simulink model "DFIG_BESS_In_power_LFnetwork_5bus"  (R2017b)
settings: Solver=ode23tb  StartTime=0.0  StopTime=10  MaxStep=0.04  RelTol=1e-3  EnableMultiTasking=on
values from neighbouring files (symbols this model uses):
  beta = beta (k)    [Parameter_2M_DFIG_BESS.m]
  Cbus = 80e-3    (= 0.08)    [Parameter_2M_DFIG_BESS.m]
  Cbus_bess = 15e-3    (= 0.015)    [Parameter_2M_DFIG_BESS.m]
  Cfilter = 80e-3    (= 0.08)    [Parameter_2M_DFIG_BESS.m]
  cp_opt_abs = abs(max(Cp))    [Parameter_2M_DFIG_BESS.m]
  D = 0.1    [Parameter_2M_DFIG_BESS.m]
  f = 60    [Parameter_2M_DFIG_BESS.m]
  Fs = 1.8    [Parameter_2M_DFIG_BESS.m]
  fsw = 4e3    (= 4000)    [Parameter_2M_DFIG_BESS.m]
  J = 90    [Parameter_2M_DFIG_BESS.m]
  ki_id = (wni^2)*Lr*sigma    (= 491.599501999)    [Parameter_2M_DFIG_BESS.m]
  ki_idg = (wnig^2)*Lg    (= 68.6450725305)    [Parameter_2M_DFIG_BESS.m]
  ki_iq = ki_id    (= 491.599501999)    [Parameter_2M_DFIG_BESS.m]
  ki_iqg = ki_idg    (= 68.6450725305)    [Parameter_2M_DFIG_BESS.m]
  ki_v = -300000    [Parameter_2M_DFIG_BESS.m]
  kp_id = (2*wni*sigma*Lr)-Rr    (= 0.5771)    [Parameter_2M_DFIG_BESS.m]
  kp_idg = (2*wnig*Lg)-Rg    (= 0.364153420404)    [Parameter_2M_DFIG_BESS.m]
  kp_iq = kp_id    (= 0.5771)    [Parameter_2M_DFIG_BESS.m]
  kp_iqg = kp_idg    (= 0.364153420404)    [Parameter_2M_DFIG_BESS.m]
  kp_v = -1000    [Parameter_2M_DFIG_BESS.m]
  Kpg = 1/(1.5*Vs*sqrt(2/3))    [Parameter_2M_DFIG_BESS.m]
  Kqg = -Kpg    [Parameter_2M_DFIG_BESS.m]
  lambda_opt = abs(lambda(posicion))    [Parameter_2M_DFIG_BESS.m]
  Lfilter = 483e-6    (= 0.000483)    [Parameter_2M_DFIG_BESS.m]
  Lg = 483e-6    (= 0.000483)    [Parameter_2M_DFIG_BESS.m]
  Lm = 2.5e-3    (= 0.0025)    [Parameter_2M_DFIG_BESS.m]
  Lr = Lm + Lsr    (= 0.002587)    [Parameter_2M_DFIG_BESS.m]
  Ls = Lm + Lsi    (= 0.002587)    [Parameter_2M_DFIG_BESS.m]
  Lsi = 87e-6    (= 8.7e-05)    [Parameter_2M_DFIG_BESS.m]
  n = 1800    [Parameter_2M_DFIG_BESS.m]
  N = 100    [Parameter_2M_DFIG_BESS.m]
  p = 2    [Parameter_2M_DFIG_BESS.m]
  Ps = 2e6    (= 2000000)    [Parameter_2M_DFIG_BESS.m]
  Radio = 44    [Parameter_2M_DFIG_BESS.m]
  Rfilter = 20e-3    (= 0.02)    [Parameter_2M_DFIG_BESS.m]
  ro = 1.225    [Parameter_2M_DFIG_BESS.m]
  Rr = 2.9e-3    (= 0.0029)    [Parameter_2M_DFIG_BESS.m]
  Rs = 2.6e-3    (= 0.0026)    [Parameter_2M_DFIG_BESS.m]
  sigma = 1- Lm^2/(Ls*Lr)    (= 0.0661284179513)    [Parameter_2M_DFIG_BESS.m]
  Vbus_ref = 1200    [Parameter_2M_DFIG_BESS.m]
  Vdc_bat_ref = 1300    [Parameter_2M_DFIG_BESS.m]
  Vs = 690    [Parameter_2M_DFIG_BESS.m]
undefined symbols (not defined in the file or in its folder): D1, Delta, DiscIntNeverNeededParam, Ion, Lithium, sigbuilder_block
libraries: powerlib x69, powerlib_meascontrol x21, electricdrivelib x1, peGeneralControl x1
(part 2 of 3)

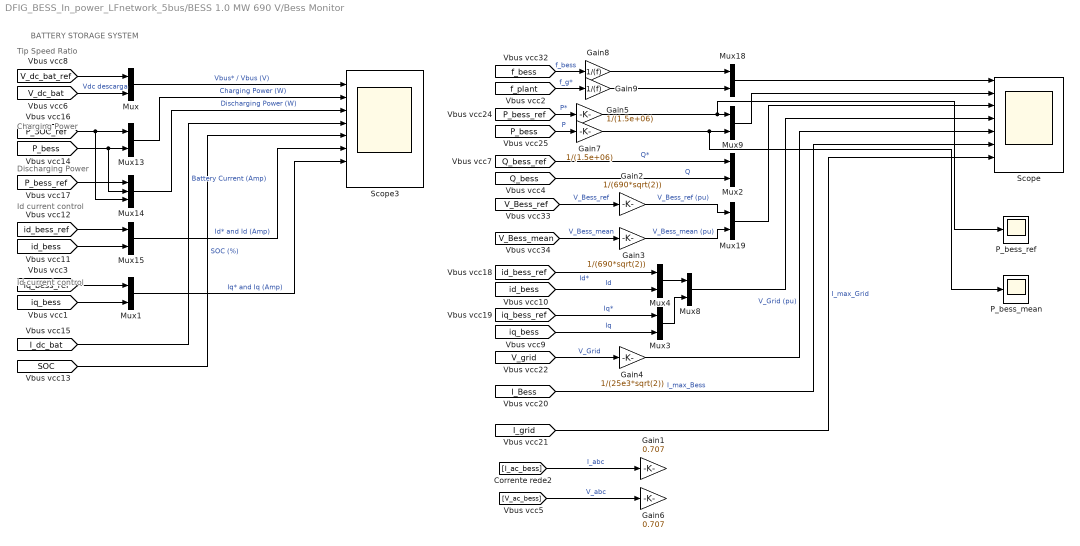
== system DFIG_BESS_In_power_LFnetwork_5bus/BESS 1.0 MW 690 V/Bess Monitor ==
  note: BATTERY STORAGE SYSTEM
  note: Tip Speed Ratio
  note: Charging Power
  note: Discharging Power
  note: Id current control
  note: Id current control
  Gain1 : Gain  Gain=0.707
  Gain2 : Gain  Gain=1/(690*sqrt(2))
  Gain3 : Gain  Gain=1/(690*sqrt(2))
  Gain4 : Gain  Gain=1/(25e3*sqrt(2))
  Gain5 : Gain  Gain=1/(1.5e+06)
  Gain6 : Gain  Gain=0.707
  Gain7 : Gain  Gain=1/(1.5e+06)
  Gain8 : Gain  Gain=1/(f)
  Gain9 : Gain  Gain=1/(f)
  Mux{,1..4,8..9,13,15,18..19} (11 alike) : Mux  Inputs=2
  Mux14 : Mux  Inputs=3
  P_bess_mean : Scope
  P_bess_ref : Scope
  Scope : Scope  NumInputPorts=8
  Scope3 : Scope  NumInputPorts=8
  wires:
  [P_bess_ref] -> Mux14/1
  Mux13/1 -> Scope3/2  "Charging Power (W)"
  [P_SOC_ref] -> Mux14/3, Mux13/1
  [P_bess] -> Mux14/2, Mux13/2
  [id_bess_ref] -> Mux15/1
  [V_dc_bat_ref] -> Mux/1
  Mux/1 -> Scope3/1  "Vbus* / Vbus (V)"
  [id_bess] -> Mux15/2
  Mux14/1 -> Scope3/3  "Discharging Power (W)"
  [SOC] -> Scope3/5  "SOC (%)"
  [I_dc_bat] -> Scope3/4  "Battery Current (Amp)"
  Mux15/1 -> Scope3/6  "Id* and Id (Amp)"
  [V_dc_bat] -> Mux/2  "Vdc descarga"
  [iq_bess] -> Mux1/2
  [iq_bess_ref] -> Mux1/1
  Mux1/1 -> Scope3/7  "Iq* and Iq (Amp)"
  [Q_bess_ref] -> Mux2/1  "Q*"
  [iq_bess_ref] -> Mux3/1  "Iq*"
  [id_bess] -> Mux4/2  "Id"
  [iq_bess] -> Mux3/2  "Iq"
  [id_bess_ref] -> Mux4/1  "Id*"
  Mux4/1 -> Mux8/1
  Mux3/1 -> Mux8/2
  [P_bess_ref] -> Gain5/1  "P*"
  [f_bess] -> Gain8/1  "f_bess"
  [f_plant] -> Gain9/1  "f_g*"
  Mux18/1 -> Scope/1
  [V_Bess_ref] -> Gain2/1  "V_Bess_ref"
  [V_Bess_mean] -> Gain3/1  "V_Bess_mean"
  [V_ac_bess] -> Gain6/1  "V_abc"
  [I_ac_bess] -> Gain1/1  "I_abc"
  [V_grid] -> Gain4/1  "V_Grid"
  [P_bess] -> Gain7/1  "P"
  [Q_bess] -> Mux2/2  "Q"
  Gain2/1 -> Mux19/1  "V_Bess_ref (pu)"
  Gain3/1 -> Mux19/2  "V_Bess_mean (pu)"
  Gain4/1 -> Scope/5  "V_Grid (pu)"
  [I_Bess] -> Scope/6  "I_max_Bess"
  [I_grid] -> Scope/7  "I_max_Grid"
  Mux9/1 -> Scope/2
  Mux19/1 -> Scope/3
  Mux8/1 -> Scope/4
  Gain5/1 -> P_bess_ref/1, Mux9/1
  Gain7/1 -> P_bess_mean/1, Mux9/2
  Gain8/1 -> Mux18/1
  Gain9/1 -> Mux18/2

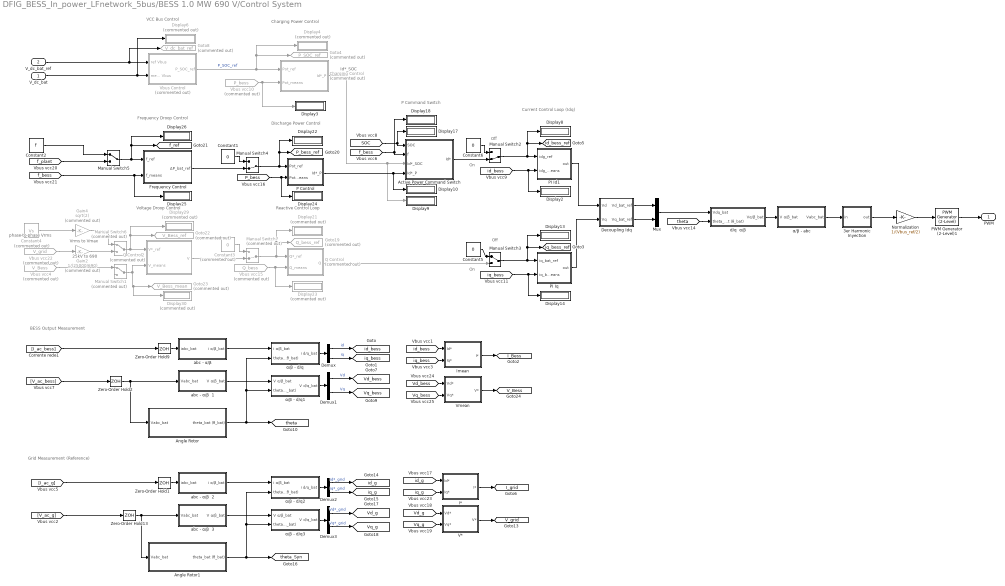
== system DFIG_BESS_In_power_LFnetwork_5bus/BESS 1.0 MW 690 V/Control System ==
  note: BESS Output Measurement
  note: Id*_SOC
  note: Grid Measurement (Reference)
  note: Current Control Loop (Idq)
  note: Discharge Power Control
  note: Frequency Droop Control
  note: Voltage Droop Control
  note: Reactive Control Loop
  note: 25kV to 690
  note: VCC Bus Control
  note: Charging Power Control
  note: P Command Switch
  note: Vrms to Vmax
  note: phase-to-phase Vrms
  note: On
  note: Off
  note: On
  note: Off
  V_dc_bat : Inport
  V_dc_bat_ref : Inport  Port=2
  " Angle Rotor" : Subsystem
  " Angle Rotor1" : Subsystem
  3er Harmonic Inyection : Subsystem
  Active Power Command Switch : Subsystem
  Charging Control : Subsystem  Commented=on
  Constant1 : Constant  Value=0
  Constant2 : Constant  Value=f
  Constant3 : Constant  Commented=on  Value=0
  Constant4 : Constant  Commented=on  Value=Vs
  Constant5 : Constant  Value=0
  Constant6 : Constant  Value=0
  Decoupling Idq : Subsystem
  Demux{,1..3} (4 alike) : Demux  Outputs=2
  Display{2..3,8..10,13..14,17..18,22,24..26} (13 alike) : Display
  Display{4,6,21,23,29..30} (6 alike) : Display  Commented=on
  Frequency Control : Subsystem
  Gain2 : Gain  Commented=on  Gain=1/(25000/690)
  Gain4 : Gain  Commented=on  Gain=sqrt(2)
  Goto19 : Goto  Commented=on  GotoTag=Q_bess_ref  TagVisibility=global
  Goto22 : Goto  Commented=on  GotoTag=V_Bess_ref  TagVisibility=global
  Goto23 : Goto  Commented=on  GotoTag=V_Bess_mean  TagVisibility=global
  Goto4 : Goto  Commented=on  GotoTag=P_SOC_ref  TagVisibility=global
  Goto8 : Goto  Commented=on  GotoTag=V_dc_bat_ref  TagVisibility=global
  I* : Subsystem
  Imean : Subsystem
  Manual Switch1 : ManualSwitch  Commented=on
  Manual Switch2 : ManualSwitch  CurrentSetting=0
  Manual Switch3 : ManualSwitch
  Manual Switch4 : ManualSwitch  CurrentSetting=0
  Manual Switch5 : ManualSwitch
  Manual Switch6 : ManualSwitch  Commented=on
  Manual Switch7 : ManualSwitch  Commented=on  CurrentSetting=0
  Mux : Mux  Inputs=2
  Normalization : Gain  Gain=1/(Vbus_ref/2)
  P Control : Subsystem
  PI Id1 : Subsystem
  PI Iq : Subsystem
  PWM Generator (2-Level)1 : powerlib_meascontrol/Pulse & Signal Generators/PWM Generator (2-Level)  ModulatorType=Three-phase bridge (6 pulses)  ModulatorMode=Unsynchronized  Fc=fsw  Pc=0  nF=27  MinMax="[ -1  1 ]"  SamplingTechnique=Natural  ModulatingSignals=off  m=0.8  Freq=60  Phase=0  Ts=0  ShowCarrierOutport=off
      settings: SourceProductName=Simscape Power Systems
  Q Control : Subsystem  Commented=on
  Q Control2 : Subsystem  Commented=on
  V* : Subsystem
  Vbus Control : Subsystem  Commented=on
  Vbus vcc10 : From  Commented=on  GotoTag=P_bess  TagVisibility=global
  Vbus vcc15 : From  Commented=on  GotoTag=Q_bess  TagVisibility=global
  Vbus vcc22 : From  Commented=on  GotoTag=V_grid  TagVisibility=global
  Vbus vcc4 : From  Commented=on  GotoTag=V_Bess  TagVisibility=global
  Vmean : Subsystem
  Zero-Order Hold{1..2,9,13} (4 alike) : ZeroOrderHold  SampleTime=1/fsw
  "abc - α/β  " : Subsystem
  abc - α/β  1 : Subsystem
  abc - α/β  2 : Subsystem
  abc - α/β  3 : Subsystem
  "d/q  α/β " : Subsystem
  α/β - abc : Subsystem
  α/β - d/q : Subsystem
  α/β - d/q1 : Subsystem
  α/β - d/q2 : Subsystem
  α/β - d/q3 : Subsystem
  PWM : Outport
  tag scope: I_Bess=global, I_grid=global, P_bess_ref=global, V_Bess=global, V_grid=global, Vd_bess=global, Vd_g=global, Vq_bess=global, Vq_g=global, f_ref=global, id_bess=global, id_bess_ref=global, id_g=global, iq_bess=global, iq_bess_ref=global, iq_g=global, theta=global, theta_Syn=global
  wires:
  PWM Generator (2-Level)1/1 -> PWM/1
  α/β - d/q/1(i d/q_bat) -> Demux/1
  Zero-Order Hold2/1 -> " Angle Rotor"/1(Vabc_bat), abc - α/β  1/1(Vabc_bat)
  α/β - abc/1(Vabc_bat) -> 3er Harmonic Inyection/1(in)
  Zero-Order Hold9/1 -> "abc - α/β  "/1(iabc_bat)
  "d/q  α/β "/1("Vα/β_bat ") -> α/β - abc/1(V α/β_bat)
  "abc - α/β  "/1(i α/β_bat) -> α/β - d/q/1(i α/β_bat)
  3er Harmonic Inyection/1(out) -> Normalization/1
  PI Id1/1(out) -> Decoupling Idq/1(Vd)
  PI Iq/1("out ") -> Decoupling Idq/2(Vq)
  Normalization/1 -> PWM Generator (2-Level)1/1
  V_dc_bat/1 -> Display6/1, Vbus Control/2("means Vbus ")
  [f_bess] -> Active Power Command Switch/2(f), Display18/1
  [SOC] -> Active Power Command Switch/1(SOC), Display17/1
  V_dc_bat_ref/1 -> Goto8/1, Vbus Control/1("ref Vbus ")
  Vbus Control/1(P_SOC_ref) -> Goto4/1, Display4/1, Charging Control/1("Pot_ref ")  "P_SOC_ref"
  Vbus vcc10/1 -> Charging Control/2("Pot_means "), Display3/1
  Demux1/1 -> [Vd_bess]  "Vd"
  abc - α/β  1/1(V α/β_bat) -> α/β - d/q1/1(V α/β_bat)
  α/β - d/q1/1(V d/q_bat) -> Demux1/1
  Demux1/2 -> [Vq_bess]  "Vq"
  Mux/1 -> "d/q  α/β "/1(Vdq_bat)
  Decoupling Idq/1(" Vd_bat_ref") -> Mux/1
  Decoupling Idq/2(" Vq_bat_ref") -> Mux/2
  " Angle Rotor"/1(theta_bat (θ_bat)) -> α/β - d/q1/2(theta_bat (θ_bat)), α/β - d/q/2(theta_bat (θ_bat)), [theta]
  Demux/1 -> [id_bess]  "id"
  Demux/2 -> [iq_bess]  "iq"
  [theta] -> "d/q  α/β "/2(theta_bat (θ_bat))
  [id_bess] -> PI Id1/2(idg_means), Display2/1
  [iq_bess] -> Display14/1, PI Iq/2(iq_bat_means)
  Demux3/2 -> [Vq_g]  "Vq*_grid"
  Demux3/1 -> [Vd_g]  "Vd*_grid"
  abc - α/β  3/1(V α/β_bat) -> α/β - d/q3/1(V α/β_bat)
  abc - α/β  2/1(i α/β_bat) -> α/β - d/q2/1(i α/β_bat)
  " Angle Rotor1"/1(theta_bat (θ_bat)) -> α/β - d/q3/2(theta_bat (θ_bat)), α/β - d/q2/2(theta_bat (θ_bat)), [theta_Syn]
  Demux2/1 -> [id_g]  "id*_grid"
  Demux2/2 -> [iq_g]  "iq*_grid"
  α/β - d/q2/1(i d/q_bat) -> Demux2/1
  α/β - d/q3/1(V d/q_bat) -> Demux3/1
  [I_ac_g] -> Zero-Order Hold1/1
  [V_ac_g] -> Zero-Order Hold13/1
  Zero-Order Hold1/1 -> abc - α/β  2/1(iabc_bat)
  Zero-Order Hold13/1 -> " Angle Rotor1"/1(Vabc_bat), abc - α/β  3/1(Vabc_bat)
  [P_bess] -> Display24/1, P Control/2("Pot_means ")
  Manual Switch2/1 -> Display8/1, [id_bess_ref], PI Id1/1(idg_ref)
  Manual Switch3/1 -> Display13/1, [iq_bess_ref], PI Iq/1(iq_bat_ref)
  [f_bess] -> Display25/1, Frequency Control/2(f_means)
  Manual Switch4/1 -> [P_bess_ref], Display22/1, P Control/1("Pot_ref ")
  Frequency Control/1("ΔP_bat_ref ") -> Manual Switch4/2
  Constant1/1 -> Manual Switch4/1
  Manual Switch5/1 -> Display26/1, [f_ref], Frequency Control/1(f_ref)
  [Vq_g] -> V*/2(Vq*)
  [Vd_g] -> V*/1(Vd*)
  [Vd_bess] -> Vmean/1(Vd*)
  [Vq_bess] -> Vmean/2(Vq*)
  Vbus vcc15/1 -> Display23/1, Q Control/2(Q_means)
  Manual Switch7/1 -> Goto19/1, Display21/1, Q Control/1(Q*_ref)
  Constant3/1 -> Manual Switch7/1
  [f_plant] -> Manual Switch5/2
  Constant2/1 -> Manual Switch5/1
  Constant5/1 -> Manual Switch3/1
  Q Control2/1("V ") -> Manual Switch7/2
  V*/1("V* ") -> [V_grid]
  Vmean/1("V* ") -> [V_Bess]
  Manual Switch6/1 -> Q Control2/1(V*_ref), Display29/1, Goto22/1
  [I_ac_bess] -> Zero-Order Hold9/1
  [V_ac_bess] -> Zero-Order Hold2/1
  Vbus vcc22/1 -> Gain2/1
  Gain2/1 -> Manual Switch6/2
  Q Control/1("Q ") -> Manual Switch3/2
  Active Power Command Switch/1(Id*) -> Manual Switch2/2
  Charging Control/1(Id*_P) -> Display9/1, Active Power Command Switch/3(Id*_SOC)
  P Control/1(Id*_P) -> Active Power Command Switch/4(Id*_P), Display10/1
  Constant4/1 -> Gain4/1
  Gain4/1 -> Manual Switch6/1
  Imean/1("I* ") -> [I_Bess]
  [iq_bess] -> Imean/2(Iq*)
  [id_bess] -> Imean/1(Id*)
  I*/1("I* ") -> [I_grid]
  [id_g] -> I*/1(Id*)
  [iq_g] -> I*/2(Iq*)
  Constant6/1 -> Manual Switch2/1
  Manual Switch1/1 -> Q Control2/2(V_means), Display30/1, Goto23/1
  Vbus vcc4/1 -> Manual Switch1/1

== system DFIG_BESS_In_power_LFnetwork_5bus/BESS 1.0 MW 690 V/Measurement of Power - Frequency ==
  FP : Fcn  Commented=on  Expr=cos(atan(u[1]/u[2]))
  Manual Switch3 : ManualSwitch
  Mux : Mux  Commented=on  Inputs=2
  PLL (3ph)1 : powerlib_meascontrol/PLL/PLL (3ph)  Commented=on  Fmin=45  Par_Init=[0, f]  ParK=[180, 3200, 1]  TcD=1e-4  MaxRateChangeFreq=12  FilterCutOffFreq=25  Ts=0  AGC=on
  "Power (3ph, Instantaneous)1" : powerlib_meascontrol/Measurements/Power (3ph, Instantaneous)
      settings: SourceProductName=Simscape Power Systems
  Scope : Scope  Commented=on
  F (Hz) : Outport
  P (W) : Outport  Port=2
  Q (VAR) : Outport  Port=3
  Angle (0) : Outport  Port=4
  tag scope: P_bess=global, Q_bess=global, f_bess=global, wt_mean=global
  wires:
  [V_ac_bess] -> "Power (3ph, Instantaneous)1"/1, PLL (3ph)1/1
  "Power (3ph, Instantaneous)1"/1 -> [P_bess], Mux/2, P (W)/1  "Pot"
  [I_ac_bess] -> "Power (3ph, Instantaneous)1"/2
  "Power (3ph, Instantaneous)1"/2 -> Mux/1, Q (VAR)/1, [Q_bess]
  PLL (3ph)1/2 -> Angle (0)/1, [wt_mean]
  Mux/1 -> FP/1
  FP/1 -> Scope/1
  [f_dfig_bess] -> Manual Switch3/1
  PLL (3ph)1/1 -> Manual Switch3/2
  Manual Switch3/1 -> F (Hz)/1, [f_bess]

== system DFIG_BESS_In_power_LFnetwork_5bus/BESS 1.0 MW 690 V/Subsystem1 ==
  In1 : Inport
  Bus Selector : BusSelector  OutputSignals=SOC (%),Current (A),Voltage (V)
  tag scope: I_dc_bat=global, SOC=global, V_dc_bat=global
  wires:
  Bus Selector/3 -> [V_dc_bat]  "<Voltage (V)>"
  Bus Selector/1 -> [SOC]  "<SOC (%)>"
  In1/1 -> Bus Selector/1
  Bus Selector/2 -> [I_dc_bat]  "<Current (A)>"

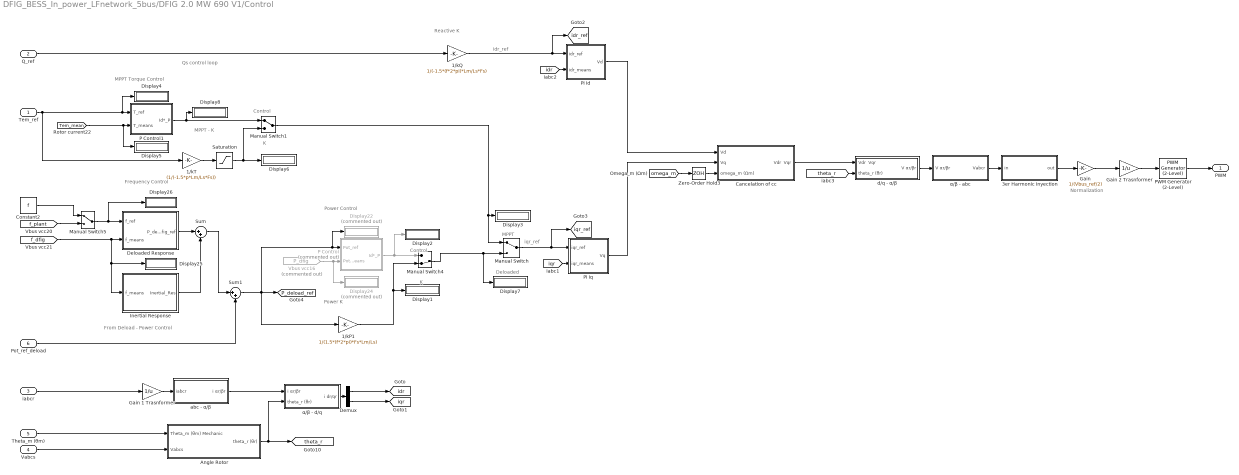
== system DFIG_BESS_In_power_LFnetwork_5bus/DFIG 2.0 MW 690 V1/Control ==
  note: Normalization
  note: iqr_ref
  note: idr_ref
  note: Qs control loop
  note: Reactive K
  note: MPPT - K
  note: From Deload - Power Control
  note: Frequency Control
  note: Power Control
  note: Power K
  note: MPPT
  note: Deloaded
  note: Control
  note: K
  note: MPPT Torque Control
  note: Control
  note: K
  Tem_ref : Inport
  Q_ref : Inport  Port=2
  iabcr : Inport  Port=3
  Vabcs : Inport  Port=4
  Theta_m (θm) : Inport  Port=5
  Pot_ref_deload : Inport  Port=6
  " Angle Rotor" : Subsystem
  1/kP1 : Gain  Gain=1/(1.5*(f*2*pi)*Fs*Lm/Ls)
  1/kQ : Gain  Gain=1/(-1.5*(f*2*pi)*Lm/Ls*Fs)
  1/kT : Gain  Gain=(1/(-1.5*p*Lm/Ls*Fs))
  3er Harmonic Inyection : Subsystem
  Cancelation of cc : Subsystem
  Constant2 : Constant  Value=f
  Deloaded Response : Subsystem
  Demux : Demux  Outputs=2
  Display{1..8,25..26} (10 alike) : Display
  Display22 : Display  Commented=on
  Display24 : Display  Commented=on
  Gain : Gain  Gain=1/(Vbus_ref/2)
  Gain 1 Trasnformer : Gain  Gain=1/u
  Gain 2 Trasnformer : Gain  Gain=1/u
  Inertial Response : Subsystem
  Manual Switch : ManualSwitch
  Manual Switch1 : ManualSwitch
  Manual Switch4 : ManualSwitch  CurrentSetting=0
  Manual Switch5 : ManualSwitch
  P Control : Subsystem  Commented=on
  P Control1 : Subsystem
  PI Id : Subsystem
  PI Iq : Subsystem
  PWM Generator (2-Level) : powerlib_meascontrol/Pulse & Signal Generators/PWM Generator (2-Level)  ModulatorType=Three-phase bridge (6 pulses)  ModulatorMode=Unsynchronized  Fc=fsw  Pc=0  nF=27  MinMax="[ -1  1 ]"  SamplingTechnique=Natural  ModulatingSignals=off  m=0.8  Freq=60  Phase=0  Ts=0  ShowCarrierOutport=off
      settings: SourceProductName=Simscape Power Systems
  Saturation : Saturate  UpperLimit=3500  LowerLimit=0
  Sum : Sum  Inputs=|++
  Sum1 : Sum  Inputs=|++
  Vbus vcc16 : From  Commented=on  GotoTag=P_dfig  TagVisibility=global
  Zero-Order Hold3 : ZeroOrderHold  SampleTime=1/fsw
  "abc - α/β " : Subsystem
  d/q - α/β : Subsystem
  α/β - abc : Subsystem
  α/β - d/q : Subsystem
  PWM : Outport
  tag scope: P_deload_ref=global, idr=global, idr_ref=global, iqr=global, iqr_ref=global, theta_r=global
  wires:
  α/β - abc/1(Vabcr) -> 3er Harmonic Inyection/1(in)
  d/q - α/β/1(V αr/βr) -> α/β - abc/1(V αr/βr)
  iabcr/1 -> Gain 1 Trasnformer/1
  "abc - α/β "/1(i αr/βr) -> α/β - d/q/1(i αr/βr)
  3er Harmonic Inyection/1(out) -> Gain/1
  Theta_m (θm)/1 -> " Angle Rotor"/1(Theta_m (θm) Mechanic)
  Vabcs/1 -> " Angle Rotor"/2(Vabcs)
  " Angle Rotor"/1(theta_r (θr)) -> [theta_r], α/β - d/q/2(theta_r (θr))
  PI Id/1(Vd) -> Cancelation of cc/1(Vd)
  PI Iq/1(Vq) -> Cancelation of cc/2(Vq)
  α/β - d/q/1(i dr/qr) -> Demux/1
  Demux/2 -> [iqr]
  Demux/1 -> [idr]
  Q_ref/1 -> 1/kQ/1
  Cancelation of cc/1(Vdr  Vqr) -> d/q - α/β/1(Vdr  Vqr)
  Gain/1 -> Gain 2 Trasnformer/1
  Gain 1 Trasnformer/1 -> "abc - α/β "/1(iabcr)
  Gain 2 Trasnformer/1 -> PWM Generator (2-Level)/1
  PWM Generator (2-Level)/1 -> PWM/1
  1/kQ/1 -> [idr_ref], PI Id/1(idr_ref)
  Manual Switch/1 -> [iqr_ref], PI Iq/1(iqr_ref)
  [idr] -> PI Id/2(idr_means)
  [iqr] -> PI Iq/2(iqr_means)
  Constant2/1 -> Manual Switch5/1
  [f_dfig] -> Inertial Response/1(f_means), Display25/1, Deloaded Response/2(f_means)
  Manual Switch5/1 -> Display26/1, Deloaded Response/1(f_ref)
  [f_plant] -> Manual Switch5/2
  [theta_r] -> d/q - α/β/2(theta_r (θr))
  [omega_m] -> Zero-Order Hold3/1
  Zero-Order Hold3/1 -> Cancelation of cc/3(omega_m (Ωm))
  Deloaded Response/1("P_deloaded_dfig_ref ") -> Sum/1
  Sum/1 -> Sum1/1
  Pot_ref_deload/1 -> Sum1/2
  Inertial Response/1("Inertial_Res ") -> Sum/2
  Vbus vcc16/1 -> Display24/1, P Control/2("Pot_means ")
  Sum1/1 -> 1/kP1/1, [P_deload_ref], Display22/1, P Control/1("Pot_ref ")
  P Control/1(Id*_P) -> Manual Switch4/1, Display2/1
  1/kP1/1 -> Display1/1, Manual Switch4/2
  Manual Switch4/1 -> Display7/1, Manual Switch/2
  1/kT/1 -> Saturation/1
  P Control1/1(Id*_P) -> Display8/1, Manual Switch1/1
  Manual Switch1/1 -> Display3/1, Manual Switch/1
  Tem_ref/1 -> Display4/1, P Control1/1("T_ref "), 1/kT/1
  [Tem_mean] -> Display5/1, P Control1/2("T_means ")
  Saturation/1 -> Display6/1, Manual Switch1/2

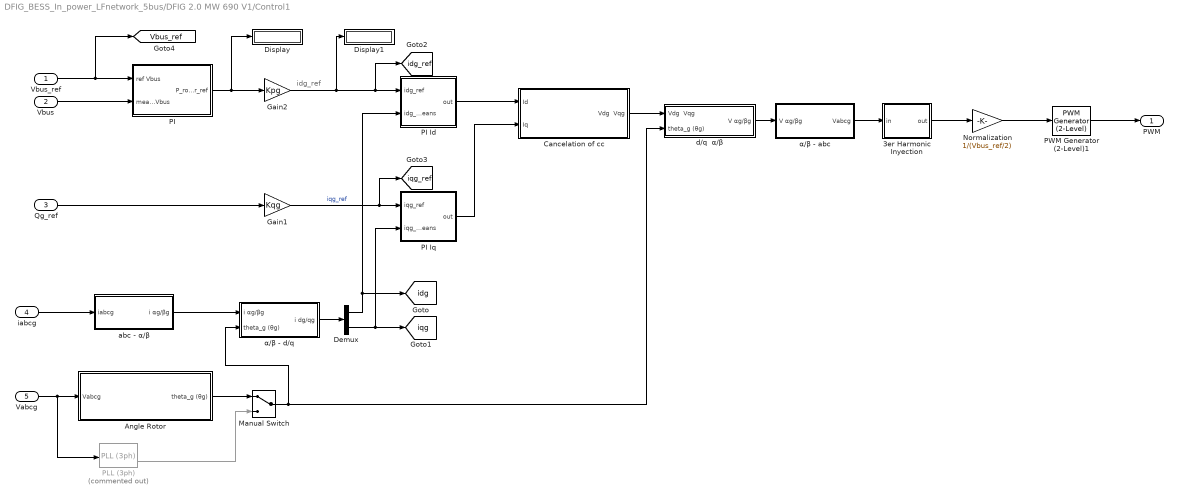
== system DFIG_BESS_In_power_LFnetwork_5bus/DFIG 2.0 MW 690 V1/Control1 ==
  note: idg_ref
  Vbus_ref : Inport
  Vbus : Inport  Port=2
  Qg_ref : Inport  Port=3
  iabcg : Inport  Port=4
  "Vabcg " : Inport  Port=5
  " Angle Rotor" : Subsystem
  3er Harmonic Inyection : Subsystem
  Cancelation of cc : Subsystem
  Demux : Demux  Outputs=2
  Display : Display
  Display1 : Display
  Gain1 : Gain  Gain=Kqg
  Gain2 : Gain  Gain=Kpg
  Manual Switch : ManualSwitch
  Normalization : Gain  Gain=1/(Vbus_ref/2)
  PI : Subsystem
  PI Id : Subsystem
  PI Iq : Subsystem
  PLL (3ph) : powerlib_meascontrol/PLL/PLL (3ph)  Commented=on  Fmin=45  Par_Init=[0, 60]  ParK=[180, 3200, 1]  TcD=1e-4  MaxRateChangeFreq=12  FilterCutOffFreq=25  Ts=0  AGC=on
      link override Model/abc to dq0: Alignment=Aligned with phase A axis
  PWM Generator (2-Level)1 : powerlib_meascontrol/Pulse & Signal Generators/PWM Generator (2-Level)  ModulatorType=Three-phase bridge (6 pulses)  ModulatorMode=Unsynchronized  Fc=fsw  Pc=0  nF=27  MinMax="[ -1  1 ]"  SamplingTechnique=Natural  ModulatingSignals=off  m=0.8  Freq=60  Phase=0  Ts=0  ShowCarrierOutport=off
      settings: SourceProductName=Simscape Power Systems
  "abc - α/β  " : Subsystem
  "d/q  α/β " : Subsystem
  α/β - abc : Subsystem
  α/β - d/q : Subsystem
  PWM : Outport
  tag scope: Vbus_ref=global, idg=global, idg_ref=global, iqg=global, iqg_ref=global
  wires:
  Normalization/1 -> PWM Generator (2-Level)1/1
  Cancelation of cc/1(Vdg  Vqg) -> "d/q  α/β "/1(Vdg  Vqg)
  Gain1/1 -> PI Iq/1(iqg_ref), [iqg_ref]  "iqg_ref"
  Demux/1 -> PI Id/2(idg_means), [idg]
  Demux/2 -> PI Iq/2(iqg_means), [iqg]
  PI Iq/1(out) -> Cancelation of cc/2(Iq)
  PI Id/1(out) -> Cancelation of cc/1(Id)
  3er Harmonic Inyection/1(out) -> Normalization/1
  "abc - α/β  "/1(i αg/βg) -> α/β - d/q/1(i αg/βg)
  "d/q  α/β "/1(V αg/βg) -> α/β - abc/1(V αg/βg)
  iabcg/1 -> "abc - α/β  "/1(iabcg)
  Vbus_ref/1 -> [Vbus_ref], PI/1("ref Vbus ")
  Gain2/1 -> Display1/1, [idg_ref], PI Id/1(idg_ref)
  Vbus/1 -> PI/2("means Vbus ")
  Qg_ref/1 -> Gain1/1
  α/β - abc/1(Vabcg) -> 3er Harmonic Inyection/1(in)
  "Vabcg "/1 -> " Angle Rotor"/1("Vabcg "), PLL (3ph)/1
  PI/1(P_rotor_ref) -> Display/1, Gain2/1
  " Angle Rotor"/1(theta_g (θg)) -> Manual Switch/1
  Manual Switch/1 -> "d/q  α/β "/2(theta_g (θg)), α/β - d/q/2(theta_g (θg))
  α/β - d/q/1(i dg/qg) -> Demux/1
  PLL (3ph)/2 -> Manual Switch/2
  PWM Generator (2-Level)1/1 -> PWM/1

== system DFIG_BESS_In_power_LFnetwork_5bus/DFIG 2.0 MW 690 V1/Deload ==
  Wind speed (m/s) : Inport
  CP : Constant  Value=0.40
  CP1 : Constant  Value=0.44
  Display1 : Display
  Display2 : Display
  Mux6 : Mux  Inputs=2
  Mux7 : Mux  Inputs=2
  Pt_deload : Fcn  Expr=0.5*ro*pi*(Radio)^2*(u[1])^3*u[2]
  Pt_max : Fcn  Expr=0.5*ro*pi*(Radio)^2*(u[1])^3*u[2]
  Scope1 : Scope  NumInputPorts=2
  Sum : Sum  Inputs=|-+
  P_deload : Outport
  P_Max : Outport  Port=2
  P_backup : Outport  Port=3
  wires:
  CP/1 -> Mux6/2
  Mux6/1 -> Pt_deload/1
  Wind speed (m/s)/1 -> Mux7/1, Mux6/1
  Mux7/1 -> Pt_max/1
  CP1/1 -> Mux7/2
  Pt_deload/1 -> Sum/1, Display2/1, Scope1/1, P_deload/1
  Pt_max/1 -> Sum/2, P_Max/1, Display1/1, Scope1/2
  Sum/1 -> P_backup/1

== system DFIG_BESS_In_power_LFnetwork_5bus/DFIG 2.0 MW 690 V1/MPPT ==
  note: Zone 2: MPPT with Vw 5 - 11
  Omega_m : Inport
  Display1 : Display
  Display2 : Display
  Display3 : Display
  Gearbox Ratio Generator Torque (-)1 : Gain  Gain=-1/N
  Gearbox Ratio1 : Gain  Gain=1/N
  Kopt : Gain  Gain=0.5*ro*pi*(Radio)^5/(lambda_opt)^3*cp_opt_abs
  Product2 : Product  Inputs=**  SaturateOnIntegerOverflow=on  InputSameDT=on  OutDataTypeStr=Inherit: Same as first input
  Saturation : Saturate  UpperLimit=2.6e+06  LowerLimit=0
  omega^2 : Fcn  Expr=(u[1])^2
  Tem_ref : Outport
  "Pot_ref " : Outport  Port=2
  wires:
  Gearbox Ratio1/1 -> Product2/2, omega^2/1
  omega^2/1 -> Kopt/1
  Kopt/1 -> Product2/1, Display3/1, Gearbox Ratio Generator Torque (-)1/1
  Product2/1 -> Saturation/1, Display1/1  "Pt"
  Gearbox Ratio Generator Torque (-)1/1 -> Display2/1, Tem_ref/1
  Omega_m/1 -> Gearbox Ratio1/1
  Saturation/1 -> "Pot_ref "/1

== system DFIG_BESS_In_power_LFnetwork_5bus/DFIG 2.0 MW 690 V1/Measurement of Power - Frequency ==
  FP : Fcn  Commented=on  Expr=cos(atan(u[1]/u[2]))
  Manual Switch3 : ManualSwitch
  Mux : Mux  Commented=on  Inputs=2
  PLL (3ph)1 : powerlib_meascontrol/PLL/PLL (3ph)  Commented=on  Fmin=45  Par_Init=[0, f]  ParK=[180, 3200, 1]  TcD=1e-4  MaxRateChangeFreq=12  FilterCutOffFreq=25  Ts=0  AGC=on
  "Power (3ph, Instantaneous)1" : powerlib_meascontrol/Measurements/Power (3ph, Instantaneous)
      settings: SourceProductName=Simscape Power Systems
  Scope : Scope  Commented=on
  F (Hz) : Outport
  P (W) : Outport  Port=2
  Q (VAR) : Outport  Port=3
  Angle (0) : Outport  Port=4
  tag scope: P_dfig=global, Q_dfig=global, f_dfig=global, wt_mean_dfig=global
  wires:
  [Vdfig] -> "Power (3ph, Instantaneous)1"/1, PLL (3ph)1/1
  "Power (3ph, Instantaneous)1"/1 -> Mux/2, P (W)/1, [P_dfig]  "Pot"
  [Idfig] -> "Power (3ph, Instantaneous)1"/2
  "Power (3ph, Instantaneous)1"/2 -> Mux/1, Q (VAR)/1, [Q_dfig]
  PLL (3ph)1/2 -> Angle (0)/1, [wt_mean_dfig]
  Mux/1 -> FP/1
  FP/1 -> Scope/1
  [f_dfig_bess] -> Manual Switch3/1
  Manual Switch3/1 -> [f_dfig], F (Hz)/1
  PLL (3ph)1/1 -> Manual Switch3/2

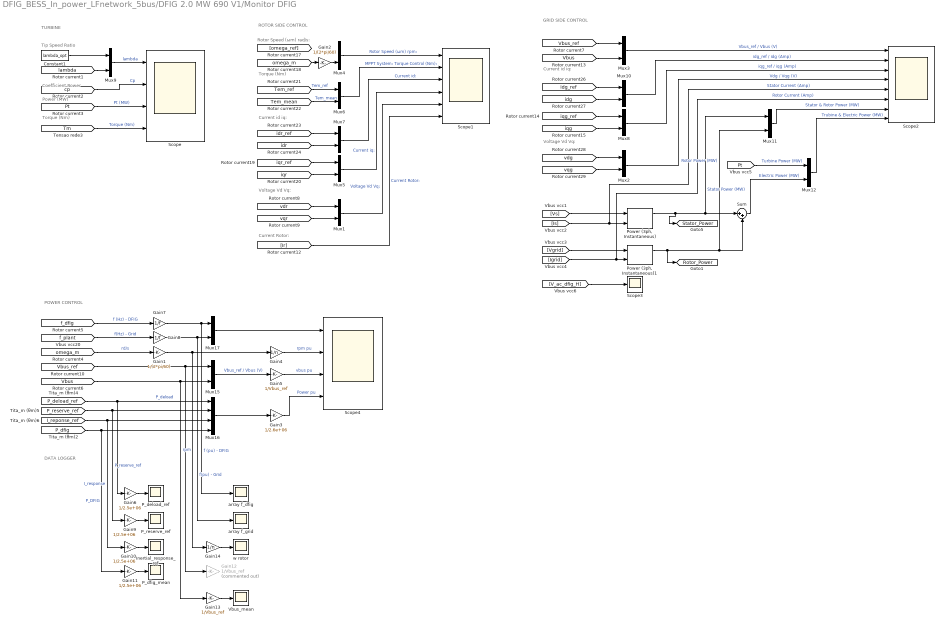
== system DFIG_BESS_In_power_LFnetwork_5bus/DFIG 2.0 MW 690 V1/Monitor DFIG ==
  note: ROTOR SIDE CONTROL
  note: Torque (Nm)
  note: Current id iq:
  note: Rotor Speed (ωm) rad/s:
  note: Voltage Vd Vq:
  note: TURBINE
  note: Torque (Nm)
  note: Power (MW)
  note: Coefficient Power
  note: Tip Speed Ratio
  note: GRID SIDE CONTROL
  note: Current id iq:
  note: Voltage Vd Vq:
  note: Current Rotor:
  note: POWER CONTROL
  note: DATA LOGGER
  Constant1 : Constant  Value=lambda_opt
  Gain1 : Gain  Gain=1/(2*pi/60)
  Gain{6,9..11} (4 alike) : Gain  Gain=1/2.5e+06
  Gain12 : Gain  Commented=on  Gain=1/Vbus_ref
  Gain13 : Gain  Gain=1/Vbus_ref
  Gain14 : Gain  Gain=1/n
  Gain2 : Gain  Gain=1/(2*pi/60)
  Gain3 : Gain  Gain=1/2.6e+06
  Gain4 : Gain  Gain=1/n
  Gain5 : Gain  Gain=1/Vbus_ref
  Gain7 : Gain  Gain=1/f
  Gain8 : Gain  Gain=1/f
  Inertial_response_ref : Scope
  Mux{1..12,15,17} (14 alike) : Mux  Inputs=2
  Mux16 : Mux
  P_deload_ref : Scope
  P_dfig_mean : Scope
  P_reserve_ref : Scope
  "Power (3ph, Instantaneous)" : powerlib_meascontrol/Measurements/Power (3ph, Instantaneous)
      settings: SourceProductName=Simscape Power Systems
  "Power (3ph, Instantaneous)1" : powerlib_meascontrol/Measurements/Power (3ph, Instantaneous)
      settings: SourceProductName=Simscape Power Systems
  Scope : Scope  NumInputPorts=4
  Scope1 : Scope  NumInputPorts=6
  Scope2 : Scope  NumInputPorts=8
  Scope3 : Scope
  Scope4 : Scope  NumInputPorts=4
  Sum : Sum  Inputs=|++
  Vbus_mean : Scope
  array f_dfig : Scope
  array f_grid : Scope
  w rotor : Scope
  tag scope: Rotor_Power=global, Stator_Power=global
  wires:
  [iqr_ref] -> Mux5/1
  [iqr] -> Mux5/2
  [idr] -> Mux7/2
  [idr_ref] -> Mux7/1
  [vdr] -> Mux1/1
  [vqr] -> Mux1/2
  [vqg] -> Mux2/2
  [vdg] -> Mux2/1
  [idg_ref] -> Mux10/1
  [idg] -> Mux10/2
  [iqg] -> Mux8/2
  [iqg_ref] -> Mux8/1
  [Tem_ref] -> Mux6/1  "Tem_ref"
  [Vbus] -> Mux3/2
  [Vbus_ref] -> Mux3/1
  [cp] -> Scope/2  "Cp"
  [Pt] -> Scope/3  "Pt (MW)"
  [Tm] -> Scope/4  "Torque (Nm)"
  Mux4/1 -> Scope1/1  "Rotor Speed (ωm) rpm:"
  Mux6/1 -> Scope1/2  "MPPT System: Torque Control (Nm):"
  Mux7/1 -> Scope1/3  "Current id:"
  Mux5/1 -> Scope1/4  "Current iq:"
  Mux1/1 -> Scope1/5  "Voltage Vd Vq:"
  [Ir] -> Scope1/6  "Current Rotor:"
  [omega_m] -> Gain2/1
  Gain2/1 -> Mux4/2
  Mux3/1 -> Scope2/1  "Vbus_ref / Vbus (V)"
  Mux10/1 -> Scope2/2  "idg_ref / idg (Amp)"
  Mux8/1 -> Scope2/3  "iqg_ref / iqg (Amp)"
  Mux2/1 -> Scope2/4  "Vdg / Vqg (V)"
  [lambda] -> Mux9/2
  Constant1/1 -> Mux9/1
  Mux9/1 -> Scope/1  "lambda"
  [Tem_mean] -> Mux6/2  "Tem_mean"
  [Vs] -> "Power (3ph, Instantaneous)"/1
  [Vgrid] -> "Power (3ph, Instantaneous)1"/1
  [Igrid] -> "Power (3ph, Instantaneous)1"/2, Scope2/6  "Rotor Current (Amp)"
  [Is] -> "Power (3ph, Instantaneous)"/2, Scope2/5  "Stator Current (Amp)"
  "Power (3ph, Instantaneous)"/1 -> [Stator_Power], Mux11/1, Sum/1  "Stator Power (MW)"
  "Power (3ph, Instantaneous)1"/1 -> [Rotor_Power], Sum/2, Mux11/2  "Rotor Power (MW)"
  Sum/1 -> Mux12/2  "Electric Power (MW)"
  Mux11/1 -> Scope2/7  "Stator & Rotor Power (MW)"
  [Pt] -> Mux12/1  "Turbine Power (MW)"
  Mux12/1 -> Scope2/8  "Trubine & Electric Power (MW)"
  [V_ac_dfig_H] -> Scope3/1
  [omega_m] -> Gain1/1  "rd/s"
  [Vbus] -> Gain13/1, Mux15/2
  [Vbus_ref] -> Gain12/1, Mux15/1
  [P_deload_ref] -> Gain6/1, Mux16/1  "P_deload"
  [P_reserve_ref] -> Gain9/1, Mux16/2  "P_reserve_ref"
  [I_reponse_ref] -> Gain10/1, Mux16/3  "I_response"
  Mux17/1 -> Scope4/1
  [f_dfig] -> Gain7/1  "f (Hz) - DFIG"
  [f_plant] -> Gain8/1  "f(Hz) - Grid"
  Gain1/1 -> Gain14/1, Gain4/1  "rpm"
  Mux15/1 -> Gain5/1  "Vbus_ref / Vbus (V)"
  [P_dfig] -> Gain11/1, Mux16/4  "P_DFIG"
  Gain4/1 -> Scope4/2  "rpm pu"
  Gain5/1 -> Scope4/3  "vbus pu"
  Mux16/1 -> Gain3/1
  Gain7/1 -> array f_dfig/1, Mux17/1  "f (pu) - DFIG"
  Gain8/1 -> array f_grid/1, Mux17/2  "f(pu) - Grid"
  Gain3/1 -> Scope4/4  "Power pu"
  Gain6/1 -> P_deload_ref/1
  Gain9/1 -> P_reserve_ref/1
  Gain10/1 -> Inertial_response_ref/1
  Gain11/1 -> P_dfig_mean/1
  Gain13/1 -> Vbus_mean/1
  Gain14/1 -> w rotor/1

== system DFIG_BESS_In_power_LFnetwork_5bus/DFIG 2.0 MW 690 V1/Signal Builder ==
  Demux : Demux  Tag=STV Demux  Outputs=1
  FromWs : FromWorkspace  Tag=STV FromWs  VariableName=tuvar  SampleTime=0
      SigBuilderData=|
      | common.afterFinalStr = 'Extrapolate'
      | common.sampleTime = 0
      | dataSet.timeRange = [0 20]
      | dataSet.name = 'Group 1'
      | sbobj.Groups.Name = 'Group 1'
      | sbobj.Groups.Signals.Name = 'Signal 1'
      | sbobj.Groups.Signals.XData = [0 1.5 4.8 5 5.2 5.44 5.7 6.08 6.5 6.84 7.18 7.62 8 8.42 8.98 9.48 10 10.4 10.88 11.36 11.8 12.32 12.88 13.38 14.1 14.74 15.28 15.86 16.32 16.86 17.5 18.1 18.62 19.32 20]
      | sbobj.Groups.Signals.YData = [0 11.5 11.5471428571 11.4 10.3 9.95 9.75 10.05 10.5 10.95 11.1 11.15 11.55 11.65 11.5 11.3 11.35 11.35 11.45 11.35 11.15 11.35 11.5 11.4859550562 11.55 11.5228813559 11.5 11.4754237288 11.4559322034 11.4330508475 11.4059322034 11.3805084746 11.3584745763 11.3288135593 11.3]
      | sbobj.Groups.TimeRange = [0 20]
  Signal 1 : Outport  Tag=STV Outport
  wires:
  Demux/1 -> Signal 1/1
  FromWs/1 -> Demux/1

== system DFIG_BESS_In_power_LFnetwork_5bus/DFIG 2.0 MW 690 V1/Signal Builder1 ==
  Demux : Demux  Tag=STV Demux  Outputs=1
  FromWs : FromWorkspace  Tag=STV FromWs  VariableName=tuvar  SampleTime=0
      SigBuilderData=|
      | common.afterFinalStr = 'Extrapolate'
      | common.sampleTime = 0
      | dataSet.timeRange = [0 20]
      | dataSet.name = 'Group 1'
      | sbobj.Groups.Name = 'Group 1'
      | sbobj.Groups.Signals.Name = 'Signal 1'
      | sbobj.Groups.Signals.XData = [0 1 2.5 3 3.2 3.44 3.7 4.08 4.5 4.84 5.18 5.62 6 6.42 6.98 7.5 8 8.5 9 9.5 10 10.5 12.88 13.38 14.1 14.74 15.28 15.86 16.32 16.86 17.5 18.1 18.62 19.32 20]
      | sbobj.Groups.Signals.YData = [0 11.5 11.5 11.5 11.38 11.5 11.56 11.41 10.73 10.57 10.7 11.04 11.38 11.62 11.25 11.44 11.62 11.65 11.45 11.35 11.38 11.35 11.5 11.4859550562 11.55 11.5228813559 11.5 11.4754237288 11.4559322034 11.4330508475 11.4059322034 11.3805084746 11.3584745763 11.3288135593 11.3]
      | sbobj.Groups.TimeRange = [0 20]
  Signal 1 : Outport  Tag=STV Outport
  wires:
  FromWs/1 -> Demux/1
  Demux/1 -> Signal 1/1

== system DFIG_BESS_In_power_LFnetwork_5bus/DFIG 2.0 MW 690 V1/Subsystem ==
  In1 : Inport
  Bus Selector : BusSelector  OutputSignals=Mechanical.Rotor angle thetam (rad),Mechanical.Rotor speed (wm),Mechanical.Electromagnetic torque Te (N*m)
  tag scope: Tem_mean=global, omega_m=global, tita_m=global
  wires:
  Bus Selector/2 -> [omega_m]  "<Rotor speed (wm)>"
  In1/1 -> Bus Selector/1
  Bus Selector/1 -> [tita_m]  "<Rotor angle thetam (rad)>"
  Bus Selector/3 -> [Tem_mean]  "<Electromagnetic torque Te (N*m)>"

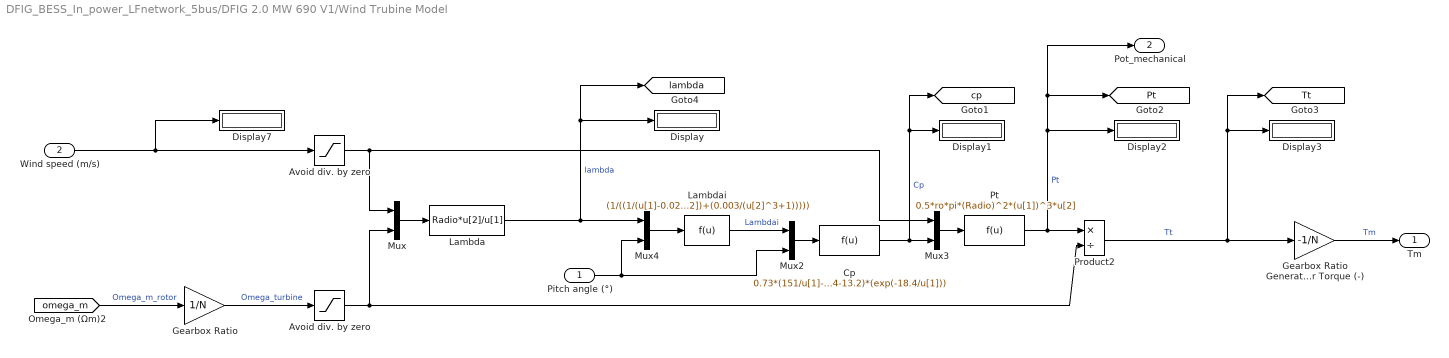
== system DFIG_BESS_In_power_LFnetwork_5bus/DFIG 2.0 MW 690 V1/Wind Trubine Model ==
  Pitch angle (°) : Inport
  Wind speed (m/s) : Inport  Port=2
  Avoid div. by zero : Saturate  UpperLimit=inf  LowerLimit=eps
  "Avoid div. by zero " : Saturate  UpperLimit=inf  LowerLimit=eps
  Cp : Fcn  Expr=0.73*(151/u[1]-0.58*u[2]-0.002*u[2]^2.14-13.2)*(exp(-18.4/u[1]))
  Display{,1..3,7} (5 alike) : Display
  Gearbox Ratio : Gain  Gain=1/N
  Gearbox Ratio Generator Torque (-) : Gain  Gain=-1/N
  Lambda : Fcn  Expr=Radio*u[2]/u[1]
  Lambdai : Fcn  Expr=(1/((1/(u[1]-0.02*u[2])+(0.003/(u[2]^3+1)))))
  Mux{,2..4} (4 alike) : Mux  Inputs=2
  Product2 : Product  Inputs=*/  SaturateOnIntegerOverflow=on  InputSameDT=on  OutDataTypeStr=Inherit: Same as first input
  Pt : Fcn  Expr=0.5*ro*pi*(Radio)^2*(u[1])^3*u[2]
  Tm : Outport
  Pot_mechanical : Outport  Port=2
  tag scope: Pt=global, Tt=global, cp=global, lambda=global
  wires:
  "Avoid div. by zero "/1 -> Product2/2, Mux/2
  Avoid div. by zero/1 -> Mux/1, Mux3/1
  [omega_m] -> Gearbox Ratio/1  "Omega_m_rotor"
  Mux3/1 -> Pt/1
  Cp/1 -> Display1/1, [cp], Mux3/2  "Cp"
  Mux/1 -> Lambda/1
  Mux2/1 -> Cp/1
  Product2/1 -> Display3/1, [Tt], Gearbox Ratio Generator Torque (-)/1  "Tt"
  Pt/1 -> Display2/1, Pot_mechanical/1, [Pt], Product2/1  "Pt"
  Gearbox Ratio/1 -> "Avoid div. by zero "/1  "Omega_turbine"
  Wind speed (m/s)/1 -> Display7/1, Avoid div. by zero/1
  Lambdai/1 -> Mux2/1  "Lambdai"
  Mux4/1 -> Lambdai/1
  Gearbox Ratio Generator Torque (-)/1 -> Tm/1  "Tm"
  Pitch angle (°)/1 -> Mux2/2, Mux4/2
  Lambda/1 -> Display/1, [lambda], Mux4/1  "lambda"

== system DFIG_BESS_In_power_LFnetwork_5bus/BESS 1.0 MW 690 V/Control System/ Angle Rotor ==
  note: V α/β_bat
  Vabc_bat : Inport
  " abc - αβ " : Subsystem
  Demux : Demux  Outputs=2
  Manual Switch : ManualSwitch
  PLL (3ph) : powerlib_meascontrol/PLL/PLL (3ph)  Commented=on  Fmin=45  Par_Init=[0, 60]  ParK=[180, 3200, 1]  TcD=1e-4  MaxRateChangeFreq=12  FilterCutOffFreq=25  Ts=0  AGC=on
      link override Model/abc to dq0: Alignment=Aligned with phase A axis
  θv=tan^(-1) (Vβ/Vα) : Trigonometry  Operator=atan2
  theta_bat (θ_bat) : Outport
  wires:
  Demux/2 -> θv=tan^(-1) (Vβ/Vα)/1
  Demux/1 -> θv=tan^(-1) (Vβ/Vα)/2
  " abc - αβ "/1("V α/β_bat ") -> Demux/1
  Vabc_bat/1 -> PLL (3ph)/1, " abc - αβ "/1(Vabc_bat)
  PLL (3ph)/2 -> Manual Switch/2
  θv=tan^(-1) (Vβ/Vα)/1 -> Manual Switch/1
  Manual Switch/1 -> theta_bat (θ_bat)/1

== system DFIG_BESS_In_power_LFnetwork_5bus/BESS 1.0 MW 690 V/Control System/ Angle Rotor1 ==
  note: V α/β_bat
  Vabc_bat : Inport
  " abc - αβ " : Subsystem
  Demux : Demux  Outputs=2
  Manual Switch : ManualSwitch
  PLL (3ph) : powerlib_meascontrol/PLL/PLL (3ph)  Commented=on  Fmin=45  Par_Init=[0, 60]  ParK=[180, 3200, 1]  TcD=1e-4  MaxRateChangeFreq=12  FilterCutOffFreq=25  Ts=0  AGC=on
      link override Model/abc to dq0: Alignment=Aligned with phase A axis
  θv=tan^(-1) (Vβ/Vα) : Trigonometry  Operator=atan2
  theta_bat (θ_bat) : Outport
  wires:
  Demux/2 -> θv=tan^(-1) (Vβ/Vα)/1
  Demux/1 -> θv=tan^(-1) (Vβ/Vα)/2
  " abc - αβ "/1("V α/β_bat ") -> Demux/1
  Vabc_bat/1 -> PLL (3ph)/1, " abc - αβ "/1(Vabc_bat)
  PLL (3ph)/2 -> Manual Switch/2
  θv=tan^(-1) (Vβ/Vα)/1 -> Manual Switch/1
  Manual Switch/1 -> theta_bat (θ_bat)/1

== system DFIG_BESS_In_power_LFnetwork_5bus/BESS 1.0 MW 690 V/Control System/3er Harmonic Inyection ==
  in : Inport
  Gain : Gain  Gain=-0.5
  MinMax : MinMax
  MinMax1 : MinMax  Function=max
  Scope : Scope
  Sum : Sum  Inputs=|++
  Sum1 : Sum  Inputs=|++
  out : Outport
  wires:
  in/1 -> Sum1/1, MinMax1/1, MinMax/1
  MinMax/1 -> Sum/1
  MinMax1/1 -> Sum/2
  Sum1/1 -> out/1
  Sum/1 -> Gain/1
  Gain/1 -> Scope/1, Sum1/2

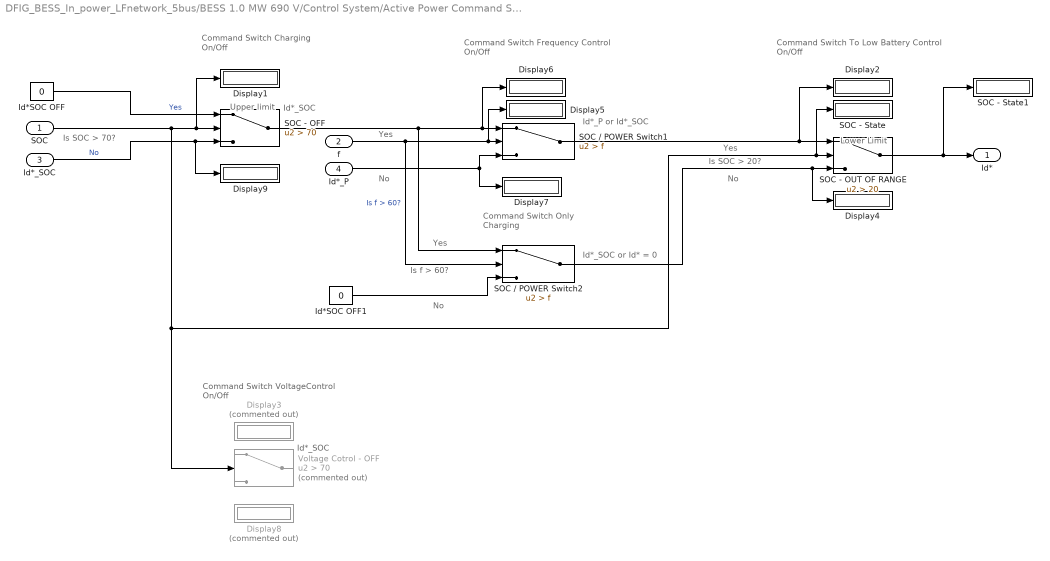
== system DFIG_BESS_In_power_LFnetwork_5bus/BESS 1.0 MW 690 V/Control System/Active Power Command Switch ==
  note: Id*_P or Id*_SOC
  note: Lower Limit
  note: Upper limit
  note: Command Switch
      | Charging On/Off
  note: Command Switch
      | Frequency Control On/Off
  note: Command Switch
      | To Low Battery Control On/Off
  note: Id*_SOC
  note: Yes
  note: Yes
  note: No
  note: Is f > 60?
  note: Yes
  note: No
  note: Command Switch
      | Only Charging
  note: No
  note: Id*_SOC or Id* = 0
  note: Is SOC > 70?
  note: Is SOC > 20?
  note: Command Switch
      | VoltageControl On/Off
  note: Id*_SOC
  SOC : Inport
  f : Inport  Port=2
  Id*_SOC : Inport  Port=3
  Id*_P : Inport  Port=4
  Display{1..2,4..7,9} (7 alike) : Display
  Display3 : Display  Commented=on
  Display8 : Display  Commented=on
  Id*SOC OFF : Constant  Value=0
  Id*SOC OFF1 : Constant  Value=0
  SOC - OFF : Switch  Criteria=u2 > Threshold  Threshold=70
  SOC - OUT OF RANGE : Switch  Criteria=u2 > Threshold  Threshold=20
  SOC - State : Display
  SOC - State1 : Display
  SOC / POWER Switch1 : Switch  Criteria=u2 > Threshold  Threshold=f
  SOC / POWER Switch2 : Switch  Criteria=u2 > Threshold  Threshold=f
  Voltage Cotrol - OFF : Switch  Commented=on  Criteria=u2 > Threshold  Threshold=70
  Id* : Outport
  wires:
  SOC / POWER Switch1/1 -> SOC - OUT OF RANGE/1, Display2/1
  f/1 -> Display5/1, SOC / POWER Switch1/2, SOC / POWER Switch2/2  "Is f > 60?"
  Id*_P/1 -> Display7/1, SOC / POWER Switch1/3
  SOC - OFF/1 -> SOC / POWER Switch1/1, Display6/1, SOC / POWER Switch2/1
  Id*_SOC/1 -> Display9/1, SOC - OFF/3  "No"
  SOC / POWER Switch2/1 -> Display4/1, SOC - OUT OF RANGE/3
  SOC - OUT OF RANGE/1 -> SOC - State1/1, Id*/1
  Id*SOC OFF1/1 -> SOC / POWER Switch2/3
  Id*SOC OFF/1 -> SOC - OFF/1  "Yes"
  SOC/1 -> SOC - State/1, SOC - OUT OF RANGE/2, Voltage Cotrol - OFF/2, Display1/1, SOC - OFF/2

== system DFIG_BESS_In_power_LFnetwork_5bus/BESS 1.0 MW 690 V/Control System/Charging Control ==
  "Pot_ref " : Inport
  "Pot_means " : Inport  Port=2
  Discrete-Time Integrator1 : DiscreteIntegrator  gainval=1  SampleTime=1/fsw  LimitOutput=on  UpperSaturationLimit=1200  LowerSaturationLimit=-1200  ICPrevOutput=DiscIntNeverNeededParam  ICPrevScaledInput=DiscIntNeverNeededParam
  Display6 : Display
  Error : Display
  Gain1 : Gain  Gain=Kpg
  Gain4 : Gain  Gain=Kpg*0.25
  Gain5 : Gain  Gain=0.03
  Mean : Display
  Mux : Mux  Inputs=3
  Ref : Display
  Sat : Display
  Sat1 : Display
  Saturation : Saturate  UpperLimit=1200  LowerLimit=-1200
  Scope : Scope
  Sum2 : Sum  Inputs=|+-
  Sum3 : Sum  Inputs=|++
  Id*_P : Outport
  wires:
  Sum2/1 -> Error/1, Mux/3, Gain5/1, Gain4/1
  Gain1/1 -> Display6/1
  Gain4/1 -> Sum3/1
  Sum3/1 -> Saturation/1
  Gain5/1 -> Discrete-Time Integrator1/1
  Discrete-Time Integrator1/1 -> Sat1/1, Sum3/2
  Mux/1 -> Scope/1
  "Pot_ref "/1 -> Mux/1, Ref/1, Gain1/1, Sum2/1
  "Pot_means "/1 -> Mux/2, Mean/1, Sum2/2
  Saturation/1 -> Sat/1, Id*_P/1

== system DFIG_BESS_In_power_LFnetwork_5bus/BESS 1.0 MW 690 V/Control System/Decoupling Idq ==
  Vd : Inport
  Vq : Inport  Port=2
  Fcn : Fcn  Expr=u[1]-u[4]*Lfilter*(2*pi*f)
  Fcn1 : Fcn  Expr=u[2]+u[3]*Lfilter*(2*pi*f)
  Mux1 : Mux
  Sum : Sum  Inputs=|++
  Sum1 : Sum  Inputs=|++
  " Vd_bat_ref" : Outport
  " Vq_bat_ref" : Outport  Port=2
  tag scope: Vd=global, Vq=global
  wires:
  Vd/1 -> Mux1/1
  Vq/1 -> Mux1/2
  Mux1/1 -> Fcn1/1, Fcn/1
  [id_bess] -> Mux1/3
  [iq_bess] -> Mux1/4
  Sum1/1 -> [Vq], " Vq_bat_ref"/1
  Fcn1/1 -> Sum1/1  "Vq*"
  Fcn/1 -> Sum/1  "Vd*"
  Sum/1 -> [Vd], " Vd_bat_ref"/1
  [Vd_bess] -> Sum/2
  [Vq_bess] -> Sum1/2

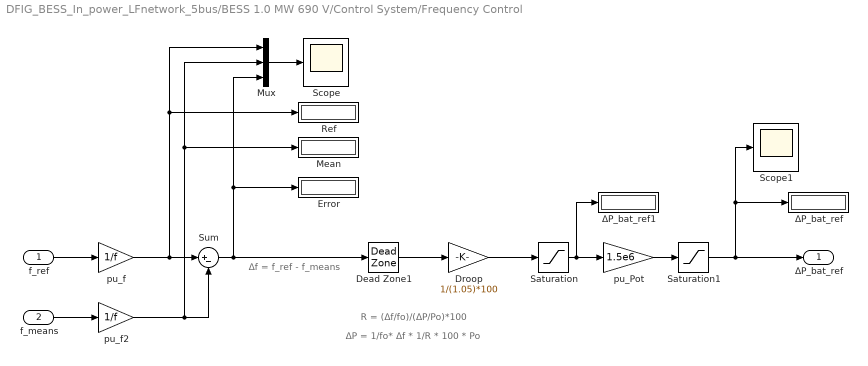
== system DFIG_BESS_In_power_LFnetwork_5bus/BESS 1.0 MW 690 V/Control System/Frequency Control ==
  note: Δf = f_ref - f_means
  note: R = (Δf/fo)/(ΔP/Po)*100
  note: ΔP = 1/fo* Δf * 1/R * 100 * Po
  f_ref : Inport
  f_means : Inport  Port=2
  Dead Zone1 : DeadZone  LowerValue=-0.00012*1/f  UpperValue=0.00002*1/f  SaturateOnIntegerOverflow=on
  Droop : Gain  Gain=1/(1.05)*100
  Error : Display
  Mean : Display
  Mux : Mux  Inputs=3
  Ref : Display
  Saturation : Saturate  UpperLimit=1  LowerLimit=0
  Saturation1 : Saturate  UpperLimit=1.5e6  LowerLimit=0
  Scope : Scope
  Scope1 : Scope
  Sum : Sum  Inputs=|+-
  "pu_Pot " : Gain  Gain=1.5e6
  pu_f : Gain  Gain=1/f
  pu_f2 : Gain  Gain=1/f
  ΔP_bat_ref : Display
  ΔP_bat_ref1 : Display
  "ΔP_bat_ref " : Outport
  wires:
  Mux/1 -> Scope/1
  f_ref/1 -> pu_f/1
  f_means/1 -> pu_f2/1
  Droop/1 -> Saturation/1
  Sum/1 -> Dead Zone1/1, Mux/3, Error/1
  Saturation/1 -> ΔP_bat_ref1/1, "pu_Pot "/1
  pu_f/1 -> Sum/1, Mux/1, Ref/1
  pu_f2/1 -> Sum/2, Mux/2, Mean/1
  "pu_Pot "/1 -> Saturation1/1
  Saturation1/1 -> Scope1/1, ΔP_bat_ref/1, "ΔP_bat_ref "/1
  Dead Zone1/1 -> Droop/1

== system DFIG_BESS_In_power_LFnetwork_5bus/BESS 1.0 MW 690 V/Control System/I* ==
  Id* : Inport
  Iq* : Inport  Port=2
  Display28 : Display
  Fcn : Fcn  Expr=sqrt((u[1])^2+(u[2])^2)
  Mux1 : Mux  Inputs=2
  "I* " : Outport
  wires:
  Fcn/1 -> Display28/1, "I* "/1
  Mux1/1 -> Fcn/1
  Id*/1 -> Mux1/1
  Iq*/1 -> Mux1/2

== system DFIG_BESS_In_power_LFnetwork_5bus/BESS 1.0 MW 690 V/Control System/Imean ==
  Id* : Inport
  Iq* : Inport  Port=2
  Display28 : Display
  Fcn : Fcn  Expr=sqrt((u[1])^2+(u[2])^2)
  Mux1 : Mux  Inputs=2
  "I* " : Outport
  wires:
  Iq*/1 -> Mux1/2
  Id*/1 -> Mux1/1
  Mux1/1 -> Fcn/1
  Fcn/1 -> Display28/1, "I* "/1

== system DFIG_BESS_In_power_LFnetwork_5bus/BESS 1.0 MW 690 V/Control System/P Control ==
  "Pot_ref " : Inport
  "Pot_means " : Inport  Port=2
  Discrete-Time Integrator1 : DiscreteIntegrator  gainval=1  SampleTime=1/fsw  LimitOutput=on  UpperSaturationLimit=1.5e6  LowerSaturationLimit=-1.5e6  ICPrevOutput=DiscIntNeverNeededParam  ICPrevScaledInput=DiscIntNeverNeededParam
  Error : Display
  Gain1 : Gain  Gain=kp_idg*1.1
  Gain4 : Gain  Gain=ki_idg*2.5
  Gain5 : Gain  Gain=Kpg
  Mean : Display
  Mux : Mux  Inputs=3
  Ref : Display
  Sat : Display
  Sat1 : Display
  Sat2 : Display
  Saturation : Saturate  UpperLimit=1.5e6  LowerLimit=-1.5e6
  Scope : Scope
  Sum2 : Sum  Inputs=|+-
  Sum3 : Sum  Inputs=|++
  Id*_P : Outport
  wires:
  Sum2/1 -> Error/1, Mux/3, Gain4/1, Gain1/1
  Gain1/1 -> Sum3/1, Sat2/1
  Sum3/1 -> Saturation/1
  Gain4/1 -> Discrete-Time Integrator1/1
  Discrete-Time Integrator1/1 -> Sat1/1, Sum3/2
  Mux/1 -> Scope/1
  "Pot_ref "/1 -> Sum2/1, Mux/1, Ref/1
  "Pot_means "/1 -> Mux/2, Mean/1, Sum2/2
  Saturation/1 -> Gain5/1, Sat/1
  Gain5/1 -> Id*_P/1

== system DFIG_BESS_In_power_LFnetwork_5bus/BESS 1.0 MW 690 V/Control System/PI Id1 ==
  idg_ref : Inport
  idg_means : Inport  Port=2
  Discrete-Time Integrator : DiscreteIntegrator  SampleTime=1/fsw  LimitOutput=on  UpperSaturationLimit=Vbus_ref/sqrt(3)*5  LowerSaturationLimit=-Vbus_ref/sqrt(3)*5  ICPrevOutput=DiscIntNeverNeededParam  ICPrevScaledInput=DiscIntNeverNeededParam
  Error : Display
  Gain : Gain  Gain=kp_idg
  Gain1 : Gain  Gain=ki_idg
  Mean : Display
  Mux : Mux  Inputs=3
  Ref : Display
  Sat : Display
  Sat 1 : Display
  Saturation : Saturate  UpperLimit=Vbus_ref/sqrt(3)*6  LowerLimit=-Vbus_ref/sqrt(3)*6
  Scope : Scope
  Sum : Sum  Inputs=|+-
  Sum1 : Sum  Inputs=|++
  out : Outport
  wires:
  Saturation/1 -> Sat/1, out/1
  Sum1/1 -> Saturation/1
  Discrete-Time Integrator/1 -> Sat 1/1, Sum1/2
  Gain1/1 -> Discrete-Time Integrator/1
  Gain/1 -> Sum1/1
  idg_means/1 -> Mean/1, Mux/2, Sum/2
  idg_ref/1 -> Ref/1, Mux/1, Sum/1
  Sum/1 -> Gain/1, Gain1/1, Mux/3, Error/1
  Mux/1 -> Scope/1

== system DFIG_BESS_In_power_LFnetwork_5bus/BESS 1.0 MW 690 V/Control System/PI Iq ==
  iq_bat_ref : Inport
  iq_bat_means : Inport  Port=2
  Discrete-Time Integrator : DiscreteIntegrator  SampleTime=1/fsw  LimitOutput=on  UpperSaturationLimit=Vbus_ref/sqrt(3)*5  LowerSaturationLimit=-Vbus_ref/sqrt(3)*5  ICPrevOutput=DiscIntNeverNeededParam  ICPrevScaledInput=DiscIntNeverNeededParam
  Error : Display
  Gain : Gain  Gain=kp_iqg
  Gain1 : Gain  Gain=ki_iqg
  Mean : Display
  Mux : Mux  Inputs=3
  Ref : Display
  Sat : Display
  Sat 1 : Display
  Saturation : Saturate  UpperLimit=Vbus_ref/sqrt(3)*6  LowerLimit=-Vbus_ref/sqrt(3)*6
  Scope : Scope
  Sum : Sum  Inputs=|+-
  Sum1 : Sum  Inputs=|++
  "out " : Outport
  wires:
  Mux/1 -> Scope/1
  Sum/1 -> Gain1/1, Gain/1, Error/1, Mux/3
  iq_bat_ref/1 -> Mux/1, Ref/1, Sum/1
  iq_bat_means/1 -> Mux/2, Mean/1, Sum/2
  Saturation/1 -> "out "/1, Sat/1
  Gain/1 -> Sum1/1
  Gain1/1 -> Discrete-Time Integrator/1
  Discrete-Time Integrator/1 -> Sum1/2, Sat 1/1
  Sum1/1 -> Saturation/1

== system DFIG_BESS_In_power_LFnetwork_5bus/BESS 1.0 MW 690 V/Control System/Q Control ==
  Q*_ref : Inport
  Q_means : Inport  Port=2
  Discrete-Time Integrator : DiscreteIntegrator  SampleTime=1/fsw  LimitOutput=on  UpperSaturationLimit=1.5e6  LowerSaturationLimit=-1.5e6  ICPrevOutput=DiscIntNeverNeededParam  ICPrevScaledInput=DiscIntNeverNeededParam
  Error : Display
  Gain1 : Gain  Gain=kp_iqg*0.25
  Gain4 : Gain  Gain=ki_iqg
  Gain5 : Gain  Gain=Kqg
  Mean : Display
  Mux : Mux  Inputs=3
  Ref : Display
  Sat : Display
  Sat 1 : Display
  Sat1 : Display
  Saturation : Saturate  UpperLimit=1.5e6  LowerLimit=-1.5e6
  Scope : Scope
  Sum : Sum  Inputs=|+-
  Sum1 : Sum  Inputs=|++
  "Q " : Outport
  wires:
  Mux/1 -> Scope/1
  Sum/1 -> Gain4/1, Gain1/1, Error/1, Mux/3
  Q*_ref/1 -> Mux/1, Ref/1, Sum/1
  Q_means/1 -> Mux/2, Mean/1, Sum/2
  Gain1/1 -> Sat1/1, Sum1/1
  Gain4/1 -> Discrete-Time Integrator/1
  Discrete-Time Integrator/1 -> Sum1/2, Sat 1/1
  Sum1/1 -> Saturation/1
  Gain5/1 -> "Q "/1
  Saturation/1 -> Gain5/1, Sat/1

== system DFIG_BESS_In_power_LFnetwork_5bus/BESS 1.0 MW 690 V/Control System/Q Control2 ==
  V*_ref : Inport
  V_means : Inport  Port=2
  Discrete-Time Integrator : DiscreteIntegrator  SampleTime=1/fsw  LimitOutput=on  UpperSaturationLimit=1.5e6  LowerSaturationLimit=-1.5e6  ICPrevOutput=DiscIntNeverNeededParam  ICPrevScaledInput=DiscIntNeverNeededParam
  Error : Display
  Gain1 : Gain  Gain=kp_iqg*1e3
  Gain4 : Gain  Gain=ki_iqg*1e3
  Mean : Display
  Mux : Mux  Inputs=3
  Ref : Display
  Sat 1 : Display
  Sat2 : Display
  Saturation : Saturate  UpperLimit=1.5e6  LowerLimit=-1.5e6
  Scope : Scope
  Sum : Sum  Inputs=|+-
  Sum1 : Sum  Inputs=|++
  "V " : Outport
  wires:
  Sum/1 -> Error/1, Mux/3, Gain4/1, Gain1/1
  Mux/1 -> Scope/1
  V*_ref/1 -> Mux/1, Ref/1, Sum/1
  V_means/1 -> Mux/2, Mean/1, Sum/2
  Gain1/1 -> Sum1/1
  Gain4/1 -> Discrete-Time Integrator/1
  Discrete-Time Integrator/1 -> Sum1/2, Sat 1/1
  Sum1/1 -> Saturation/1
  Saturation/1 -> "V "/1, Sat2/1

== system DFIG_BESS_In_power_LFnetwork_5bus/BESS 1.0 MW 690 V/Control System/V* ==
  Vd* : Inport
  Vq* : Inport  Port=2
  Display28 : Display
  Fcn : Fcn  Expr=sqrt((u[1])^2+(u[2])^2)
  Mux1 : Mux  Inputs=2
  "V* " : Outport
  wires:
  Vq*/1 -> Mux1/2
  Vd*/1 -> Mux1/1
  Mux1/1 -> Fcn/1
  Fcn/1 -> "V* "/1, Display28/1

== system DFIG_BESS_In_power_LFnetwork_5bus/BESS 1.0 MW 690 V/Control System/Vbus Control ==
  note: signal
  note: reference
  "ref Vbus " : Inport
  "means Vbus " : Inport  Port=2
  Discrete-Time Integrator1 : DiscreteIntegrator  SampleTime=1/fsw  LimitOutput=on  UpperSaturationLimit=0.5e6  LowerSaturationLimit=-0.5e6  ICPrevOutput=DiscIntNeverNeededParam  ICPrevScaledInput=DiscIntNeverNeededParam
  Error : Display
  Gain2 : Gain  Gain=-1000
  Gain3 : Gain  Gain=-300000
  Mean : Display
  Mux : Mux  Inputs=3
  Ref : Display
  Sat : Display
  Sat 1 : Display
  Saturation1 : Saturate  UpperLimit=0.4e6  LowerLimit=-0.4e6
  Scope : Scope
  Sum2 : Sum  Inputs=|+-
  Sum3 : Sum  Inputs=|++
  P_SOC_ref : Outport
  wires:
  Discrete-Time Integrator1/1 -> Sat 1/1, Sum3/2
  Gain3/1 -> Discrete-Time Integrator1/1
  Sum3/1 -> Saturation1/1
  Gain2/1 -> Sum3/1
  Saturation1/1 -> Sat/1, P_SOC_ref/1
  "means Vbus "/1 -> Sum2/2, Mean/1, Mux/2
  "ref Vbus "/1 -> Sum2/1, Ref/1, Mux/1
  Sum2/1 -> Gain2/1, Gain3/1, Mux/3, Error/1
  Mux/1 -> Scope/1

== system DFIG_BESS_In_power_LFnetwork_5bus/BESS 1.0 MW 690 V/Control System/Vmean ==
  Vd* : Inport
  Vq* : Inport  Port=2
  Display28 : Display
  Fcn : Fcn  Expr=sqrt((u[1])^2+(u[2])^2)
  Mux1 : Mux  Inputs=2
  "V* " : Outport
  wires:
  Fcn/1 -> "V* "/1, Display28/1
  Mux1/1 -> Fcn/1
  Vd*/1 -> Mux1/1
  Vq*/1 -> Mux1/2

== system DFIG_BESS_In_power_LFnetwork_5bus/BESS 1.0 MW 690 V/Control System/abc - α//β   ==
  note: iβ_bat
  note: iα_bat
  iabc_bat : Inport
  Fcn : Fcn  Expr=2/3*(u[1]-u[2]/2-u[3]/2)
  Fcn1 : Fcn  Expr=2/3*(u[2]*(sqrt(3)/2)-u[3]*(sqrt(3)/2))
  Mux : Mux  Inputs=2
  i α/β_bat : Outport
  wires:
  Mux/1 -> i α/β_bat/1
  iabc_bat/1 -> Fcn1/1, Fcn/1
  Fcn/1 -> Mux/1
  Fcn1/1 -> Mux/2

== system DFIG_BESS_In_power_LFnetwork_5bus/BESS 1.0 MW 690 V/Control System/abc - α//β  1 ==
  note: iα_bat
  note: iβ_bat
  Vabc_bat : Inport
  Fcn : Fcn  Expr=2/3*(u[1]-u[2]/2-u[3]/2)
  Fcn1 : Fcn  Expr=2/3*(u[2]*(sqrt(3)/2)-u[3]*(sqrt(3)/2))
  Mux : Mux  Inputs=2
  V α/β_bat : Outport
  wires:
  Fcn1/1 -> Mux/2
  Fcn/1 -> Mux/1
  Vabc_bat/1 -> Fcn/1, Fcn1/1
  Mux/1 -> V α/β_bat/1

== system DFIG_BESS_In_power_LFnetwork_5bus/BESS 1.0 MW 690 V/Control System/abc - α//β  2 ==
  note: iβ_bat
  note: iα_bat
  iabc_bat : Inport
  Fcn : Fcn  Expr=2/3*(u[1]-u[2]/2-u[3]/2)
  Fcn1 : Fcn  Expr=2/3*(u[2]*(sqrt(3)/2)-u[3]*(sqrt(3)/2))
  Mux : Mux  Inputs=2
  i α/β_bat : Outport
  wires:
  Mux/1 -> i α/β_bat/1
  iabc_bat/1 -> Fcn1/1, Fcn/1
  Fcn/1 -> Mux/1
  Fcn1/1 -> Mux/2

== system DFIG_BESS_In_power_LFnetwork_5bus/BESS 1.0 MW 690 V/Control System/abc - α//β  3 ==
  note: iα_bat
  note: iβ_bat
  Vabc_bat : Inport
  Fcn : Fcn  Expr=2/3*(u[1]-u[2]/2-u[3]/2)
  Fcn1 : Fcn  Expr=2/3*(u[2]*(sqrt(3)/2)-u[3]*(sqrt(3)/2))
  Mux : Mux  Inputs=2
  V α/β_bat : Outport
  wires:
  Fcn1/1 -> Mux/2
  Fcn/1 -> Mux/1
  Vabc_bat/1 -> Fcn/1, Fcn1/1
  Mux/1 -> V α/β_bat/1

== system DFIG_BESS_In_power_LFnetwork_5bus/BESS 1.0 MW 690 V/Control System/d//q  α//β  ==
  Vdq_bat : Inport
  theta_bat (θ_bat) : Inport  Port=2
  Fcn : Fcn  Expr=u(1)*cos(u[3])-u[2]*sin(u[3])
  Fcn1 : Fcn  Expr=u(1)*sin(u[3])+u[2]*cos(u[3])
  Mux : Mux  Inputs=2
  Mux1 : Mux  Inputs=2
  "Vα/β_bat " : Outport
  wires:
  Mux/1 -> "Vα/β_bat "/1
  Fcn/1 -> Mux/1
  Fcn1/1 -> Mux/2
  Vdq_bat/1 -> Mux1/1
  theta_bat (θ_bat)/1 -> Mux1/2
  Mux1/1 -> Fcn/1, Fcn1/1

== system DFIG_BESS_In_power_LFnetwork_5bus/BESS 1.0 MW 690 V/Control System/α//β - abc ==
  V α/β_bat : Inport
  Fcn : Fcn  Expr=u(1)
  Fcn1 : Fcn  Expr=-(u[1]/2)+u[2]*(sqrt(3)/2)
  Fcn2 : Fcn  Expr=-(u[1]/2)-u[2]*(sqrt(3)/2)
  Mux : Mux  Inputs=3
  Vabc_bat : Outport
  wires:
  Mux/1 -> Vabc_bat/1
  V α/β_bat/1 -> Fcn2/1, Fcn1/1, Fcn/1
  Fcn/1 -> Mux/1
  Fcn1/1 -> Mux/2
  Fcn2/1 -> Mux/3

== system DFIG_BESS_In_power_LFnetwork_5bus/BESS 1.0 MW 690 V/Control System/α//β - d//q ==
  i α/β_bat : Inport
  theta_bat (θ_bat) : Inport  Port=2
  Fcn : Fcn  Expr=u(1)*cos(u[3])+u[2]*sin(u[3])
  Fcn1 : Fcn  Expr=-u(1)*sin(u[3])+u[2]*cos(u[3])
  Mux : Mux  Inputs=2
  Mux1 : Mux  Inputs=2
  i d/q_bat : Outport
  wires:
  Mux/1 -> i d/q_bat/1
  Fcn/1 -> Mux/1
  Fcn1/1 -> Mux/2
  i α/β_bat/1 -> Mux1/1
  theta_bat (θ_bat)/1 -> Mux1/2
  Mux1/1 -> Fcn1/1, Fcn/1

== system DFIG_BESS_In_power_LFnetwork_5bus/BESS 1.0 MW 690 V/Control System/α//β - d//q1 ==
  V α/β_bat : Inport
  theta_bat (θ_bat) : Inport  Port=2
  Fcn : Fcn  Expr=u(1)*cos(u[3])+u[2]*sin(u[3])
  Fcn1 : Fcn  Expr=-u(1)*sin(u[3])+u[2]*cos(u[3])
  Mux : Mux  Inputs=2
  Mux1 : Mux  Inputs=2
  V d/q_bat : Outport
  wires:
  Mux1/1 -> Fcn/1, Fcn1/1
  theta_bat (θ_bat)/1 -> Mux1/2
  V α/β_bat/1 -> Mux1/1
  Fcn1/1 -> Mux/2
  Fcn/1 -> Mux/1
  Mux/1 -> V d/q_bat/1

== system DFIG_BESS_In_power_LFnetwork_5bus/BESS 1.0 MW 690 V/Control System/α//β - d//q2 ==
  i α/β_bat : Inport
  theta_bat (θ_bat) : Inport  Port=2
  Fcn : Fcn  Expr=u(1)*cos(u[3])+u[2]*sin(u[3])
  Fcn1 : Fcn  Expr=-u(1)*sin(u[3])+u[2]*cos(u[3])
  Mux : Mux  Inputs=2
  Mux1 : Mux  Inputs=2
  i d/q_bat : Outport
  wires:
  Mux/1 -> i d/q_bat/1
  Fcn/1 -> Mux/1
  Fcn1/1 -> Mux/2
  i α/β_bat/1 -> Mux1/1
  theta_bat (θ_bat)/1 -> Mux1/2
  Mux1/1 -> Fcn1/1, Fcn/1

== system DFIG_BESS_In_power_LFnetwork_5bus/BESS 1.0 MW 690 V/Control System/α//β - d//q3 ==
  V α/β_bat : Inport
  theta_bat (θ_bat) : Inport  Port=2
  Fcn : Fcn  Expr=u(1)*cos(u[3])+u[2]*sin(u[3])
  Fcn1 : Fcn  Expr=-u(1)*sin(u[3])+u[2]*cos(u[3])
  Mux : Mux  Inputs=2
  Mux1 : Mux  Inputs=2
  V d/q_bat : Outport
  wires:
  Mux1/1 -> Fcn/1, Fcn1/1
  theta_bat (θ_bat)/1 -> Mux1/2
  V α/β_bat/1 -> Mux1/1
  Fcn1/1 -> Mux/2
  Fcn/1 -> Mux/1
  Mux/1 -> V d/q_bat/1
